simulink model "simscape_16_nodes_projection"  (R2022b)
settings: Solver=VariableStepAuto  StartTime=0.0  StopTime=0.1  RelTol=1e-3
values from neighbouring files (symbols this model uses):
  fuzhu_ini = x_ini(1:N)    [stepchange_timevarying_change_initial_document.m]
  lambda_ini = zeros(N*(BN+N+1),1)    [stepchange_timevarying_change_initial_document.m]
  Lineindex1 = zeros(BN,2)    [stepchange_timevarying_change_initial_document.m]
  Lineindex2 = zeros(BN,3)    [stepchange_timevarying_change_initial_document.m]
  LoadI = [30.0;15.0;30.0;26.0;         18.9;22.8;29.6;32.1;         22.6;27.6;16.5;19.9;         26.5;19.4;22.7;24.9]    [stepchange_timevarying_change_initial_document.m]
  LoadZ = diag([16.7;50.0;16.7;20.0;              25.0;16.0;14.2;29.4;              18.5;19.6;22.6;25.6;              23.4;26.4;25.2;33.7])    [stepchange_timevarying_change_initial_document.m]
  nu_ini = [-0.00758212493845042	-0.0182492317603708	0.00714905390846842	0.0186908981861182          -0.00758212493845042	-0.0182492317603708	0.00714905390846842	0.0186908981861182          -0.00758212493845042	-0.0182492317603708	0.00714905390846842	0.0186908981861182          -0.00758212493845042	-0.0182492317603708	0.00714905390846842	0.0186908981861182]'    [stepchange_timevarying_change_initial_document.m]
  theta_ini = zeros(N*(BN+N+1),1)    [stepchange_timevarying_change_initial_document.m]
  u_ini = [378.9289  380.4146  379.7396  379.2243  380.1955  381.1042         379.9247  379.8974  380.0252  380.4045  379.6763  379.8341         380.1194  380.5682  379.3881  379.9696]'    [stepchange_timevarying_change_initial_document.m]
  x_hat_ini = [14.515064754915	3.95935897697232	32.9787419273847	14.9071228299889             37.6257931691129	61.1095883901259	41.4721611959256	33.6364102939300             44.9867290171943	52.8132621486412	28.1355733315040	33.0707668633162             36.6024320622732	49.3936276267038	2.38033527987224	36.4476162672594             378.638597580330	380.343321138855	379.211948658584	379.000752058610              ...(+639 chars)    [stepchange_timevarying_change_initial_document.m]
libraries: fl_lib x204, nesl_utility x101, spspowerguiLib x1
(part 1 of 3)
settings Model: Creator=27843  LastModifiedBy=27843

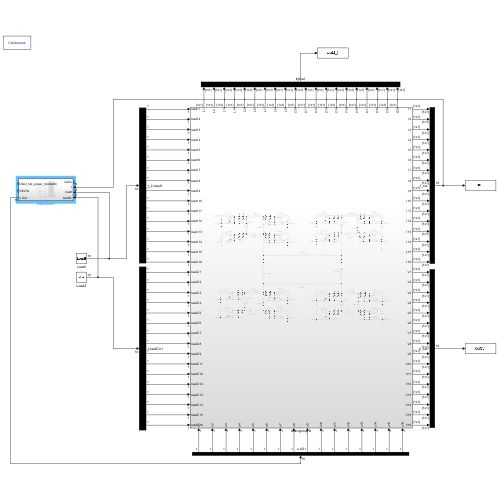
[thumbnail: Simulink's stored preview of the top-level diagram]
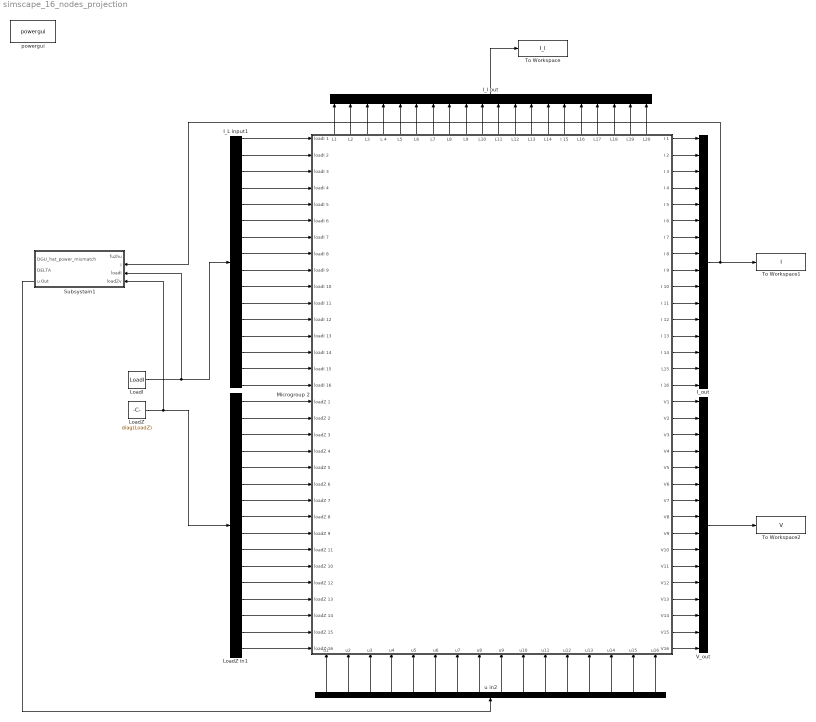
== system simscape_16_nodes_projection ==
  I_L input1 : Demux  Outputs=16
  I_l out : Mux  Inputs=20
  I_out : Mux  Inputs=16
  LoadI : Constant  Value=LoadI
  LoadZ : Constant  Value=diag(LoadZ)
  LoadZ in1 : Demux  Outputs=16
  Microgroup 2 : Subsystem
      settings: PortSchema="{\"entries\":[{\"content\":{\"sides\":[{\"content\":{\"connectorIds\":[\"In1\",\"In2\",\"In3\",\"In4\",\"In5\",\"In6\",\"In7\",\"In8\",\"In9\",\"In10\",\"In11\",\"In12\",\"In13\",\"In14\",\"In15\",\"In16\",\"In17\",\"In18\",\"In19\",\"In20\",\"In21\",\"In22\",\"In23\",\"In24\",\"In25\",\"In26\",\"In27\",\"In28\",\"In29\",\"In30\",\"In31\",\"In32\"]},\"type\":\"ConnectorPlacement.EquallySpacedRectSide\",\"uuid\":\"5197c103-f2ba-4766-bfa6-4a0cc7f0bec5\"},{\"content\":{\"connectorIds\":[\"Out1\",\"Out2\",\"Out3\",\"Out4\",\"Out5\",\"Out6\",\"Out7\",\"Out8\",\"Out9\",\"Out10\",\"Out11\",\"Out12\",\"Out13\",\"Out14\",\"Out15\",\"Out16\",\"Out17\",\"Out18\",\"Out19\",\"Out20\",\"Out21\",\"Out22\",\"Out23\",\"Out24\",\"Out25\",\"Out26\",\"Out27\",\"Out28\",\"Out29\",\"Out30\",\"Out31\",\"Out32\"],\"side\":\"RIGHT\"},\"type\":\"ConnectorPlacement.EquallySpacedRectSide\",\"uuid\":\"ba025e7b-74df-45b1-bd36-fda7dce05c8b\"},{\"content\":{\"connectorIds\":[\"Out33\",\"Out34\",\"Out35\",\"Out36\",\"Out37\",\"Out38\",\"Out39\",\"Out40\",\"Out41\",\"Out42\",\"Out43\",\"Out44\",\"Out45\",\"Out46\",\"Out47\",\"Out48\",\"Out49\",\"Out50\",\"Out51\",\"Out52\"],\"side\":\"TOP\"},\"type\":\"ConnectorPlacement.EquallySpacedRectSide\",\"uuid\":\"dfd18da5-92fe-4a7e-b123-7afeb0c6288e\"},{\"content\":{\"connectorIds\":[\"In33\",\"In34\",\"In35\",\"In36\",\"In37\",\"In38\",\"In39\",\"In40\",\"In41\",\"In42\",\"In43\",\"In44\",\"In45\",\"In46\",\"In47\",\"In48\"],\"side\":\"BOTTOM\"},\"type\":\"ConnectorPlacement.EquallySpacedRectSide\",\"uuid\":\"4fc94a7b-b545-462f-a2bc-f323440eee72\"}]},\"type\":\"ConnectorPlacement.EquallySpacedConnector\",\"uuid\":\"219570b3-6360-4866-bc3b-b38745c510e3\"}],\"packageUris\":[\"http://schema.mathworks.com/mf0/Connector/R2020b\"],\"version\":\"1.0\"}"
  Subsystem1 : Subsystem
  To Workspace : ToWorkspace  VariableName=I_l  SaveFormat=Timeseries  SampleTime=-1
  To Workspace1 : ToWorkspace  VariableName=I  SaveFormat=Timeseries  SampleTime=-1
  To Workspace2 : ToWorkspace  VariableName=V  SaveFormat=Timeseries  SampleTime=-1
  V_out : Mux  Inputs=16
  powergui : spspowerguiLib/powergui  Priority=1  SimulationMode=Continuous  SampleTime=50e-6  frequency=60  Iterations=50  frequencyindice=60  Pbase=100e6  ErrMax=1e-4  UnitsV=kV  UnitsW=MW  buscounter=0  FunctionMessages=off  echomessages=off  EnableUseOfTLC=off  CurrentSourceSwitches=off  DisableSnubberDevices=off  DisableRonSwitches=off  DisableVfSwitches=off  DisplayEquations=off  AutomaticDiscreteSolvers=off  SolverType=Tustin/Backward Euler (TBE)  Interpol=off  ExternalGateDelay=off  methode=off  Ts=100  x0status=blocks  SPID=on  SwTol=0  HookPort=off  NonlinearTolerance=1e-4  nMaxIteration=100  ContinueOnMaxIteration=off  RestoreLinks=warning  ResistiveCurrentMeasurement=off  Frange=[0:2:500]  Ylog=off  Xlog=on  ShowGrid=off  save=off  variable=ZData  structure=0  ZoomFFT=off  StartTime=0.0  cycles=1  DisplayStyle=1  fundamental=60  FreqAxis=off  MaxFrequency=1000  frequencyindicesteady=1  RmsSteady=1  display=off
  u in2 : Demux  Outputs=16
  wires:
  I_L input1/1 -> Microgroup 2/1(loadI 1)
  I_L input1/2 -> Microgroup 2/2(loadI 2)
  I_L input1/3 -> Microgroup 2/3(loadI 3)
  I_L input1/4 -> Microgroup 2/4(loadI 4)
  I_L input1/5 -> Microgroup 2/5(loadI 5)
  I_L input1/6 -> Microgroup 2/6(loadI 6)
  I_L input1/7 -> Microgroup 2/7(loadI 7)
  I_L input1/8 -> Microgroup 2/8(loadI 8)
  I_L input1/9 -> Microgroup 2/9(loadI 9)
  I_L input1/10 -> Microgroup 2/10(loadI 10)
  I_L input1/11 -> Microgroup 2/11(loadI 11)
  I_L input1/12 -> Microgroup 2/12(loadI 12)
  I_L input1/13 -> Microgroup 2/13(loadI 13)
  I_L input1/14 -> Microgroup 2/14(loadI 14)
  I_L input1/15 -> Microgroup 2/15(loadI 15)
  I_L input1/16 -> Microgroup 2/16(loadI 16)
  LoadZ in1/1 -> Microgroup 2/17(loadZ 1)
  LoadZ in1/2 -> Microgroup 2/18(loadZ 2)
  LoadZ in1/3 -> Microgroup 2/19(loadZ 3)
  LoadZ in1/4 -> Microgroup 2/20(loadZ 4)
  LoadZ in1/5 -> Microgroup 2/21(loadZ 5)
  LoadZ in1/6 -> Microgroup 2/22(loadZ 6)
  LoadZ in1/7 -> Microgroup 2/23(loadZ 7)
  LoadZ in1/8 -> Microgroup 2/24(loadZ 8)
  LoadZ in1/9 -> Microgroup 2/25(loadZ 9)
  LoadZ in1/10 -> Microgroup 2/26(loadZ 11)
  LoadZ in1/11 -> Microgroup 2/27(loadZ 10)
  LoadZ in1/12 -> Microgroup 2/28(loadZ 12)
  LoadZ in1/13 -> Microgroup 2/29(loadZ 13)
  LoadZ in1/14 -> Microgroup 2/30(loadZ 14)
  LoadZ in1/15 -> Microgroup 2/31(loadZ 15)
  LoadZ in1/16 -> Microgroup 2/32(loadZ 16)
  Microgroup 2/1(I 1) -> I_out/1
  Microgroup 2/2(I 2) -> I_out/2
  Microgroup 2/3(I 3) -> I_out/3
  Microgroup 2/4(I 4) -> I_out/4
  Microgroup 2/5(I 5) -> I_out/5
  Microgroup 2/6(I 6) -> I_out/6
  Microgroup 2/7(I 7) -> I_out/7
  Microgroup 2/8(I 8) -> I_out/8
  Microgroup 2/9(I 9) -> I_out/9
  Microgroup 2/10(I 10) -> I_out/10
  Microgroup 2/11(I 11) -> I_out/11
  Microgroup 2/12(I 12) -> I_out/12
  Microgroup 2/13(I 13) -> I_out/13
  Microgroup 2/14(I 14) -> I_out/14
  Microgroup 2/15(L15) -> I_out/15
  Microgroup 2/16(I 16) -> I_out/16
  Microgroup 2/17(V1) -> V_out/1
  Microgroup 2/18(V2) -> V_out/2
  Microgroup 2/19(V3) -> V_out/3
  Microgroup 2/20(V4) -> V_out/4
  Microgroup 2/21(V5) -> V_out/5
  Microgroup 2/22(V6) -> V_out/6
  Microgroup 2/23(V7) -> V_out/7
  Microgroup 2/24(V8) -> V_out/8
  Microgroup 2/25(V9) -> V_out/9
  Microgroup 2/26(V10) -> V_out/10
  Microgroup 2/27(V11) -> V_out/11
  Microgroup 2/28(V12) -> V_out/12
  Microgroup 2/29(V13) -> V_out/13
  Microgroup 2/30(V14) -> V_out/14
  Microgroup 2/31(V15) -> V_out/15
  Microgroup 2/32(V16) -> V_out/16
  Microgroup 2/33(L1) -> I_l out/1
  Microgroup 2/34("L2 ") -> I_l out/2
  Microgroup 2/35(L3) -> I_l out/3
  Microgroup 2/36(L 4) -> I_l out/4
  Microgroup 2/37(L5) -> I_l out/5
  Microgroup 2/38(L6) -> I_l out/6
  Microgroup 2/39(" L7") -> I_l out/7
  Microgroup 2/40(L8) -> I_l out/8
  Microgroup 2/41(L9) -> I_l out/9
  Microgroup 2/42(L10) -> I_l out/10
  Microgroup 2/43(" L11") -> I_l out/11
  Microgroup 2/44(L12) -> I_l out/12
  Microgroup 2/45(L13) -> I_l out/13
  Microgroup 2/46(L14) -> I_l out/14
  Microgroup 2/47(I 15) -> I_l out/15
  Microgroup 2/48(L16) -> I_l out/16
  Microgroup 2/49(L17) -> I_l out/17
  Microgroup 2/50(L18) -> I_l out/18
  Microgroup 2/51(L19) -> I_l out/19
  Microgroup 2/52(L20) -> I_l out/20
  u in2/1 -> Microgroup 2/33(u1)
  u in2/2 -> Microgroup 2/34(u2)
  u in2/3 -> Microgroup 2/35(u3)
  u in2/4 -> Microgroup 2/36(u4)
  u in2/5 -> Microgroup 2/37(u5)
  u in2/6 -> Microgroup 2/38(u6)
  u in2/7 -> Microgroup 2/39(u7)
  u in2/8 -> Microgroup 2/40(u8)
  u in2/9 -> Microgroup 2/41(u9)
  u in2/10 -> Microgroup 2/42(u10)
  u in2/11 -> Microgroup 2/43(u11)
  u in2/12 -> Microgroup 2/44(u12)
  u in2/13 -> Microgroup 2/45(u13)
  u in2/14 -> Microgroup 2/46(u14)
  u in2/15 -> Microgroup 2/47(u15)
  u in2/16 -> Microgroup 2/48(u16)
  Subsystem1/3(u Out) -> u in2/1
  I_out/1 -> To Workspace1/1, Subsystem1/2(I)
  LoadI/1 -> Subsystem1/3(loadI), I_L input1/1
  LoadZ/1 -> Subsystem1/4(loadZv), LoadZ in1/1
  I_l out/1 -> To Workspace/1
  V_out/1 -> To Workspace2/1
